simulink model "Sensors"  (R2017b)
settings: Solver=FixedStepDiscrete  StartTime=0.0  StopTime=10.0  FixedStep=Ts  RelTol=1e-3
settings Model: Creator=zht  LastModifiedBy=zht

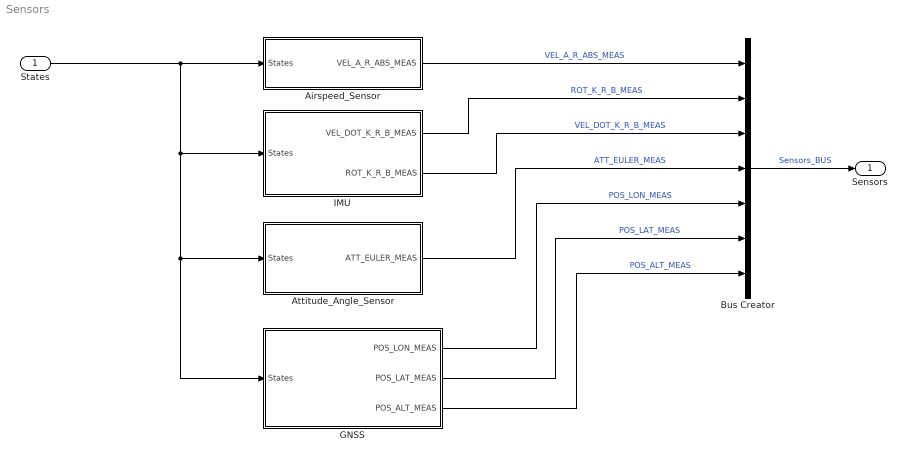
== system Sensors ==
  States : Inport  OutDataTypeStr=Bus: States_BUS
  Airspeed_Sensor : Subsystem
  "Attitude_Angle_Sensor " : Subsystem
  Bus Creator : BusCreator  Inputs=7
  "GNSS " : Subsystem
  IMU : Subsystem
  Sensors : Outport  OutDataTypeStr=Bus: Sensors_BUS
  wires:
  Bus Creator/1 -> Sensors/1  "Sensors_BUS"
  States/1 -> "Attitude_Angle_Sensor "/1(States), "GNSS "/1(States), IMU/1(States), Airspeed_Sensor/1(States)
  Airspeed_Sensor/1(VEL_A_R_ABS_MEAS) -> Bus Creator/1  "VEL_A_R_ABS_MEAS"
  IMU/1(VEL_DOT_K_R_B_MEAS) -> Bus Creator/2  "ROT_K_R_B_MEAS"
  IMU/2(ROT_K_R_B_MEAS) -> Bus Creator/3  "VEL_DOT_K_R_B_MEAS"
  "Attitude_Angle_Sensor "/1(ATT_EULER_MEAS) -> Bus Creator/4  "ATT_EULER_MEAS"
  "GNSS "/3(POS_ALT_MEAS) -> Bus Creator/7  "POS_ALT_MEAS"
  "GNSS "/2(POS_LAT_MEAS) -> Bus Creator/6  "POS_LAT_MEAS"
  "GNSS "/1(POS_LON_MEAS) -> Bus Creator/5  "POS_LON_MEAS"

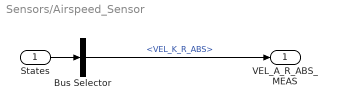
== system Sensors/Airspeed_Sensor ==
  States : Inport  OutDataTypeStr=Bus: States_BUS
  Bus Selector : BusSelector  OutputSignals=VEL_K_R_ABS
  VEL_A_R_ABS_MEAS : Outport
  wires:
  States/1 -> Bus Selector/1
  Bus Selector/1 -> VEL_A_R_ABS_MEAS/1  "<VEL_K_R_ABS>"

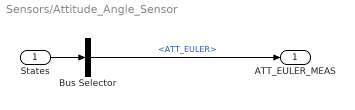
== system Sensors/Attitude_Angle_Sensor  ==
  States : Inport  OutDataTypeStr=Bus: States_BUS
  Bus Selector : BusSelector  OutputSignals=ATT_EULER
  ATT_EULER_MEAS : Outport
  wires:
  States/1 -> Bus Selector/1
  Bus Selector/1 -> ATT_EULER_MEAS/1  "<ATT_EULER>"

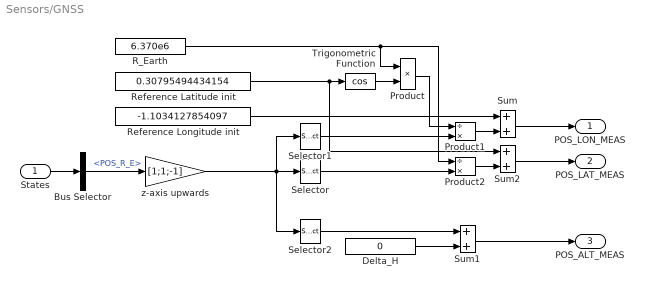
== system Sensors/GNSS  ==
  States : Inport  OutDataTypeStr=Bus: States_BUS
  Bus Selector : BusSelector  OutputSignals=POS_R_E
  Delta_H : Constant  Value=0
  Product : Product
  Product1 : Product  Inputs=/*
  Product2 : Product  Inputs=/*
  R_Earth : Constant  Value=6.370e6
  Reference Latitude init : Constant  Value=0.30795494434154
  Reference Longitude init : Constant  Value=-1.1034127854097
  Selector : Selector  InputPortWidth=3  IndexOptions=Index vector (dialog)  Indices=[1]  OutputSizes=1
  Selector1 : Selector  InputPortWidth=3  IndexOptions=Index vector (dialog)  Indices=[2]  OutputSizes=1
  Selector2 : Selector  InputPortWidth=3  IndexOptions=Index vector (dialog)  Indices=[3]  OutputSizes=1
  Sum : Sum
  Sum1 : Sum
  Sum2 : Sum
  Trigonometric Function : Trigonometry  Operator=cos
  z-axis upwards : Gain  Gain=[1;1;-1]
  POS_LON_MEAS : Outport
  POS_LAT_MEAS : Outport  Port=2
  POS_ALT_MEAS : Outport  Port=3
  wires:
  States/1 -> Bus Selector/1
  Bus Selector/1 -> z-axis upwards/1  "<POS_R_E>"
  Product/1 -> Product1/1
  Sum1/1 -> POS_ALT_MEAS/1
  Sum2/1 -> POS_LAT_MEAS/1
  Sum/1 -> POS_LON_MEAS/1
  Reference Latitude init/1 -> Trigonometric Function/1, Sum2/1
  Delta_H/1 -> Sum1/2
  R_Earth/1 -> Product2/1, Product/1
  Reference Longitude init/1 -> Sum/1
  Product2/1 -> Sum2/2
  Selector1/1 -> Product1/2
  Selector2/1 -> Sum1/1
  Product1/1 -> Sum/2
  Trigonometric Function/1 -> Product/2
  Selector/1 -> Product2/2
  z-axis upwards/1 -> Selector2/1, Selector1/1, Selector/1

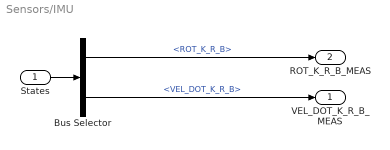
== system Sensors/IMU ==
  States : Inport  OutDataTypeStr=Bus: States_BUS
  Bus Selector : BusSelector  OutputSignals=ROT_K_R_B,VEL_DOT_K_R_B
  VEL_DOT_K_R_B_MEAS : Outport
  ROT_K_R_B_MEAS : Outport  Port=2
  wires:
  States/1 -> Bus Selector/1
  Bus Selector/1 -> ROT_K_R_B_MEAS/1  "<ROT_K_R_B>"
  Bus Selector/2 -> VEL_DOT_K_R_B_MEAS/1  "<VEL_DOT_K_R_B>"
